simulink model "ADCS_GNC_Real_Simulation"  (R2025a)
settings: Solver=ode4  StartTime=0.0  StopTime=600  FixedStep=dt_sim  RelTol=1e-3
values from neighbouring files (symbols this model uses):
  Area_drag = 1.5    [ADCS_Real_Baseline.m]    (also in ADCS_Real_Baseline_Aerospace_Toolbox.m)
  Cd = 2.2    [ADCS_Real_Baseline.m]    (also in ADCS_Real_Baseline_Aerospace_Toolbox.m)
  cp_cg_offset_drag = [0.05; 0.02; -0.03]    [ADCS_Real_Baseline.m]    (also in ADCS_Real_Baseline_Aerospace_Toolbox.m)
  g0 = 9.80665    [ADCS_Real_Baseline.m]    (also in ADCS_Real_Baseline_Aerospace_Toolbox.m)
  gyro_bias_true = [1e-4; -2e-4; 1.5e-4]    [ADCS_Real_Baseline.m]    (also in ADCS_Real_Baseline_Aerospace_Toolbox.m)
  gyro_noise_sigma = 1e-5    (= 1e-05)    [ADCS_Real_Baseline.m]    (also in ADCS_Real_Baseline_Aerospace_Toolbox.m)
  I_inv = inv(I_tensor)    [ADCS_Real_Baseline.m]    (also in ADCS_Real_Baseline_Aerospace_Toolbox.m)
  I_tensor = diag([I_xx, I_yy, I_zz])    [ADCS_Real_Baseline.m]    (also in ADCS_Real_Baseline_Aerospace_Toolbox.m)
  Kd = diag(diag(2 * zeta * I_tensor * omega_n))    [ADCS_Real_Baseline.m]    (also in ADCS_Real_Baseline_Aerospace_Toolbox.m)
  Kp = diag(diag(I_tensor * omega_n^2))    [ADCS_Real_Baseline.m]    (also in ADCS_Real_Baseline_Aerospace_Toolbox.m)
  mtq_max_dipole = 15.0    (= 15)    [ADCS_Real_Baseline.m]    (also in ADCS_Real_Baseline_Aerospace_Toolbox.m)
  mtq_power_W_per_Am2 = 0.5    [ADCS_Real_Baseline.m]    (also in ADCS_Real_Baseline_Aerospace_Toolbox.m)
  mu_E = 398600.4418    [ADCS_Real_Baseline.m]    (also in ADCS_Real_Baseline_Aerospace_Toolbox.m)
  omega_init = C_BL_init * omega_orb_LVLH    [ADCS_Real_Baseline.m]    (also in ADCS_Real_Baseline_Aerospace_Toolbox.m)
  omega_orb_mag = sqrt(mu_E / r_orbit^3)    [ADCS_Real_Baseline.m]    (also in ADCS_Real_Baseline_Aerospace_Toolbox.m)
  q_init = q_init / norm(q_init)    [ADCS_Real_Baseline.m]    (also in ADCS_Real_Baseline_Aerospace_Toolbox.m)
  q_LVLH_ECI_init = q_LVLH_ECI_init / norm(q_LVLH_ECI_init)    [ADCS_Real_Baseline.m]    (also in ADCS_Real_Baseline_Aerospace_Toolbox.m)
  r_orbit = R_E + h_orbit    (= 7171)    [ADCS_Real_Baseline.m]    (also in ADCS_Real_Baseline_Aerospace_Toolbox.m)
  rho_atm = 1e-13    [ADCS_Real_Baseline.m]    (also in ADCS_Real_Baseline_Aerospace_Toolbox.m)
  rw_max_torque = 0.05    [ADCS_Real_Baseline.m]    (also in ADCS_Real_Baseline_Aerospace_Toolbox.m)
  rw_power_W_per_Nm = 50.0    (= 50)    [ADCS_Real_Baseline.m]    (also in ADCS_Real_Baseline_Aerospace_Toolbox.m)
  st_noise_sigma = 5e-4    (= 0.0005)    [ADCS_Real_Baseline.m]    (also in ADCS_Real_Baseline_Aerospace_Toolbox.m)
  thruster_arm = 0.5    [ADCS_Real_Baseline.m]    (also in ADCS_Real_Baseline_Aerospace_Toolbox.m)
  thruster_Isp = 65.0    (= 65)    [ADCS_Real_Baseline.m]    (also in ADCS_Real_Baseline_Aerospace_Toolbox.m)
  thruster_max_torque = thruster_force * thruster_arm    (= 0.5)    [ADCS_Real_Baseline.m]    (also in ADCS_Real_Baseline_Aerospace_Toolbox.m)
  V_orb = sqrt(mu_E*1e9 / (r_orbit*1e3))    [ADCS_Real_Baseline.m]    (also in ADCS_Real_Baseline_Aerospace_Toolbox.m)
(part 2 of 2)

== matlab function ADCS_GNC_Real_Simulation/Guidance Block ==
  data: t input; q_ref output; omega_orb_mag input; omega_ref output
function [q_ref, omega_ref] = guidance_generator(t, omega_orb_mag)
% =========================================================================
% GUIDANCE & REFERENCE GENERATOR
% =========================================================================
% Purpose:
%   Generate the desired spacecraft attitude and angular velocity.
%
% Mission:
%   Smooth slew from nadir-pointing attitude to an off-nadir attitude.
%
% Reference frames:
%   ECI  = Earth-Centered Inertial frame
%   LVLH = Local Vertical Local Horizontal frame
%   BODY = Spacecraft body frame
%
% Quaternion convention:
%   q = [qw; qx; qy; qz]  (scalar first)
%
% Important convention:
%   q_ref represents the desired BODY orientation with respect to ECI.
%
%   omega_ref is the desired angular velocity of BODY with respect
%   to ECI, but EXPRESSED IN BODY COORDINATES.
%
% =========================================================================
% -------------------------------------------------------------------------
% 1. MANEUVER PARAMETERS
% -------------------------------------------------------------------------
% Time at which the maneuver starts
t_start = 10.0;                         % [s]
% Duration of the maneuver
t_duration = 120.0;                     % [s]
% Final desired attitude with respect to LVLH
roll_target  = deg2rad(30.0);            % [rad]
pitch_target = deg2rad(45.0);            % [rad]
yaw_target   = deg2rad(20.0);            % [rad]
% -------------------------------------------------------------------------
% 2. QUINTIC S-CURVE MANEUVER PROFILE
% -------------------------------------------------------------------------
% alpha goes from 0 to 1.
%
% The quintic polynomial:
%
%   alpha = 10*tau^3 - 15*tau^4 + 6*tau^5
%
% provides:
%   alpha(0) = 0
%   alpha(1) = 1
%   d_alpha(0) = 0
%   d_alpha(1) = 0
%
% Therefore the maneuver starts and ends smoothly.
if t < t_start
    % -------------------------------------------------------------
    % Phase 1: Initial attitude
    % -------------------------------------------------------------
    alpha   = 0.0;
    d_alpha = 0.0;
elseif t <= (t_start + t_duration)
    % -------------------------------------------------------------
    % Phase 2: Slew maneuver
    % -------------------------------------------------------------
    
    % Normalized maneuver time
    tau = (t - t_start) / t_duration;
    % Quintic S-curve
    alpha = 10*tau^3 - 15*tau^4 + 6*tau^5;
    % Derivative of quintic profile
    d_alpha = ...
        (30*tau^2 - 60*tau^3 + 30*tau^4) / t_duration;
else
    % -------------------------------------------------------------
    % Phase 3: Final attitude
    % -------------------------------------------------------------
    alpha   = 1.0;
    d_alpha = 0.0;
end
% -------------------------------------------------------------------------
% 3. CURRENT DESIRED EULER ANGLES
% -------------------------------------------------------------------------
% 3-2-1 / ZYX Euler sequence:
%
%   Roll  = phi
%   Pitch = theta
%   Yaw   = psi
phi   = alpha * roll_target;
theta = alpha * pitch_target;
psi   = alpha * yaw_target;
% -------------------------------------------------------------------------
% 4. EULER ANGLE RATES
% -------------------------------------------------------------------------
% Derivatives of the commanded Euler angles.
d_phi   = d_alpha * roll_target;
d_theta = d_alpha * pitch_target;
d_psi   = d_alpha * yaw_target;
% -------------------------------------------------------------------------
% 5. EULER RATES -> BODY ANGULAR VELOCITY (RIGOROUS 3-2-1 TRANSFORMATION)
% -------------------------------------------------------------------------
% IMPORTANT:
% Euler angle time derivatives (d_phi, d_theta, d_psi) are NOT body rates.
% They must be mapped into the spacecraft Body frame using the 3-2-1 kinematic matrix.
%
% omega_rel is the angular velocity of BODY relative to LVLH,
% expressed in BODY coordinates [rad/s].
omega_rel = [ ...
    d_phi - sin(theta)*d_psi;
    cos(phi)*d_theta + sin(phi)*cos(theta)*d_psi;
   -sin(phi)*d_theta + cos(phi)*cos(theta)*d_psi ];
% -------------------------------------------------------------------------
% 6. EULER ANGLES -> RELATIVE QUATERNION
% -------------------------------------------------------------------------
% Quaternion describing BODY orientation relative to LVLH.
%
% Quaternion convention:
%   q_BL = [qw; qx; qy; qz]
%
% Euler sequence:
%   ZYX / 3-2-1
cy = cos(psi * 0.5);
sy = sin(psi * 0.5);
cp = cos(theta * 0.5);
sp = sin(theta * 0.5);
cr = cos(phi * 0.5);
sr = sin(phi * 0.5);
% Quaternion BODY/LVLH
q_BL = [ ...
    cr*cp*cy + sr*sp*sy;
    sr*cp*cy - cr*sp*sy;
    cr*sp*cy + sr*cp*sy;
    cr*cp*sy - sr*sp*cy ];
% -------------------------------------------------------------------------
% 7. INITIAL LVLH ORIENTATION WITH RESPECT TO ECI
% -------------------------------------------------------------------------
% Initial LVLH-to-ECI orientation.
q_LI_init = [sqrt(2)/2;
             0;
             sqrt(2)/2;
             0];
% -------------------------------------------------------------------------
% 8. ORBITAL ROTATION
% -------------------------------------------------------------------------
% LVLH rotates with the orbit around its Y-axis.
theta_orb = -omega_orb_mag * t;
% Quaternion representing the orbital rotation around LVLH Y-axis
q_orb_rot = [ ...
    cos(theta_orb/2);
    0;
    sin(theta_orb/2);
    0 ];
% -------------------------------------------------------------------------
% 9. CURRENT LVLH ORIENTATION WITH RESPECT TO ECI
% -------------------------------------------------------------------------
% Hamilton quaternion product:
%   q_LI_curr = q_orb_rot * q_LI_init
q_LI_curr = [ ...
    q_orb_rot(1)*q_LI_init(1) ...
        - q_orb_rot(2)*q_LI_init(2) ...
        - q_orb_rot(3)*q_LI_init(3) ...
        - q_orb_rot(4)*q_LI_init(4);
    q_orb_rot(1)*q_LI_init(2) ...
        + q_orb_rot(2)*q_LI_init(1) ...
        + q_orb_rot(3)*q_LI_init(4) ...
        - q_orb_rot(4)*q_LI_init(3);
    q_orb_rot(1)*q_LI_init(3) ...
        - q_orb_rot(2)*q_LI_init(4) ...
        + q_orb_rot(3)*q_LI_init(1) ...
        + q_orb_rot(4)*q_LI_init(2);
    q_orb_rot(1)*q_LI_init(4) ...
        + q_orb_rot(2)*q_LI_init(3) ...
        - q_orb_rot(3)*q_LI_init(2) ...
        + q_orb_rot(4)*q_LI_init(1) ];
% -------------------------------------------------------------------------
% 10. DESIRED ABSOLUTE QUATERNION
% -------------------------------------------------------------------------
% Composition:
%   q_ref = q_BL * q_LI_curr
% Gives the desired BODY attitude with respect to ECI.
q_ref = [ ...
    q_BL(1)*q_LI_curr(1) ...
        - q_BL(2)*q_LI_curr(2) ...
        - q_BL(3)*q_LI_curr(3) ...
        - q_BL(4)*q_LI_curr(4);
    q_BL(1)*q_LI_curr(2) ...
        + q_BL(2)*q_LI_curr(1) ...
        + q_BL(3)*q_LI_curr(4) ...
        - q_BL(4)*q_LI_curr(3);
    q_BL(1)*q_LI_curr(3) ...
        - q_BL(2)*q_LI_curr(4) ...
        + q_BL(3)*q_LI_curr(1) ...
        + q_BL(4)*q_LI_curr(2);
    q_BL(1)*q_LI_curr(4) ...
        + q_BL(2)*q_LI_curr(3) ...
        - q_BL(3)*q_LI_curr(2) ...
        + q_BL(4)*q_LI_curr(1) ];
% -------------------------------------------------------------------------
% 11. DCM: LVLH -> BODY
% -------------------------------------------------------------------------
% Direction Cosine Matrix from LVLH coordinates to BODY coordinates.
C_BL = [ ...
    cp*cy, ...
    cp*sy, ...
   -sp;
    sr*sp*cy - cr*sy, ...
    sr*sp*sy + cr*cy, ...
    sr*cp;
    cr*sp*cy + sr*sy, ...
    cr*sp*sy - sr*cy, ...
    cr*cp ];
% -------------------------------------------------------------------------
% 12. ORBITAL ANGULAR VELOCITY
% -------------------------------------------------------------------------
omega_LVLH = [ ...
    0;
   -omega_orb_mag;
    0 ];
% -------------------------------------------------------------------------
% 13. DESIRED BODY ANGULAR VELOCITY
% -------------------------------------------------------------------------
% omega_ref = omega_body/LVLH (in body) + C_BL * omega_LVLH/ECI (in body)
% IMPORTANT: omega_ref is expressed in BODY coordinates.
omega_ref = omega_rel + C_BL * omega_LVLH;
end

== matlab function ADCS_GNC_Real_Simulation/Sensor Model_1 ==
  settings: updateMethod=DISCRETE
  data: q_true input; q_meas output; omega_true input; st_noise_sigma input; gyro_noise_sigma input; gyro_bias input; omega_meas output
function [q_meas, omega_meas] = sensor_model(q_true, omega_true, st_noise_sigma, gyro_noise_sigma, gyro_bias)
    % =====================================================================
    % SENSOR MODEL (STAR TRACKER & GYROSCOPES)
    % Inputs:
    %   q_true           : 4x1 True attitude quaternion from dynamics
    %   omega_true       : 3x1 True angular velocity from dynamics [rad/s]
    %   st_noise_sigma   : Scalar, Star Tracker noise standard deviation [rad]
    %   gyro_noise_sigma : Scalar, Gyroscope noise standard deviation [rad/s]
    %   gyro_bias        : 3x1 Gyroscope constant thermal drift [rad/s]
    %
    % Outputs:
    %   q_meas           : 4x1 Measured (noisy) quaternion
    %   omega_meas       : 3x1 Measured (noisy) angular velocity
    % =====================================================================

    % 1. GYROSCOPE MODEL (Angular Velocity)
    % Equation: w_meas = w_true + bias + noise
    % We use randn(3,1) to generate normally distributed Gaussian white noise.
    gyro_noise = gyro_noise_sigma * randn(3, 1);
    omega_meas = omega_true + gyro_bias + gyro_noise;

    % 2. STAR TRACKER MODEL (Attitude Quaternion)
    % Instead of adding noise directly to quaternion components (which breaks 
    % its properties), we generate a small random error rotation vector.
    
    % Small angle error on 3 axes [rad]
    err_angles = st_noise_sigma * randn(3, 1);
    
    % Convert small angle error to an error quaternion (Small Angle Approximation)
    % q_err = [1; theta_x/2; theta_y/2; theta_z/2]
    q_err = [1; 0.5 * err_angles(1); 0.5 * err_angles(2); 0.5 * err_angles(3)];
    q_err = q_err / norm(q_err); % Normalize just to be safe
    
    % Apply the error rotation to the true quaternion (Hamilton product)
    % q_meas = q_true * q_err
    qw = q_true(1); qx = q_true(2); qy = q_true(3); qz = q_true(4);
    ew = q_err(1);  ex = q_err(2);  ey = q_err(3);  ez = q_err(4);
    
    q_meas = [ ...
        qw*ew - qx*ex - qy*ey - qz*ez;
        qw*ex + qx*ew + qy*ez - qz*ey;
        qw*ey - qx*ez + qy*ew + qz*ex;
        qw*ez + qx*ey - qy*ex + qz*ew ];
        
    % Final normalization to ensure the controller receives a valid unit quaternion
    q_meas = q_meas / norm(q_meas);
end

== matlab function ADCS_GNC_Real_Simulation/Environment_1 ==
  data: q_BI input; torque_dist output; t input; omega_orb_mag input; q_LVLH_ECI_init input; I_tensor input; mu_E input; r_orbit input; rho_atm input; Cd input; Area_drag input; V_orb input; cp_cg_offset_drag input
function torque_dist = environment_model(q_BI, t, omega_orb_mag, q_LVLH_ECI_init, I_tensor, mu_E, r_orbit, rho_atm, Cd, Area_drag, V_orb, cp_cg_offset_drag)
    % =====================================================================
    % ENVIRONMENTAL DISTURBANCES MODEL
    % Calculates Gravity Gradient and Aerodynamic Drag torques in BODY frame.
    % =====================================================================
    
    % 1. Calculate current LVLH to ECI quaternion (Orbit evolution)
    theta_orb = -omega_orb_mag * t;
    q_orb_rot = [cos(theta_orb/2); 0; sin(theta_orb/2); 0];
    
    % Hamilton product: q_LI_curr = q_orb_rot * q_LVLH_ECI_init
    qw1 = q_orb_rot(1); qx1 = q_orb_rot(2); qy1 = q_orb_rot(3); qz1 = q_orb_rot(4);
    qw2 = q_LVLH_ECI_init(1); qx2 = q_LVLH_ECI_init(2); qy2 = q_LVLH_ECI_init(3); qz2 = q_LVLH_ECI_init(4);
    q_LI_curr = [ ...
        qw1*qw2 - qx1*qx2 - qy1*qy2 - qz1*qz2;
        qw1*qx2 + qx1*qw2 + qy1*qz2 - qz1*qy2;
        qw1*qy2 - qx1*qz2 + qy1*qw2 + qz1*qx2;
        qw1*qz2 + qx1*qy2 - qy1*qx2 + qz1*qw2 ];
        
    % 2. Calculate BODY to LVLH quaternion: q_BL = q_BI * q_LI_curr^(-1)
    q_LI_conj = [q_LI_curr(1); -q_LI_curr(2); -q_LI_curr(3); -q_LI_curr(4)];
    
    qw1 = q_BI(1); qx1 = q_BI(2); qy1 = q_BI(3); qz1 = q_BI(4);
    qw2 = q_LI_conj(1); qx2 = q_LI_conj(2); qy2 = q_LI_conj(3); qz2 = q_LI_conj(4);
    q_BL = [ ...
        qw1*qw2 - qx1*qx2 - qy1*qy2 - qz1*qz2;
        qw1*qx2 + qx1*qw2 + qy1*qz2 - qz1*qy2;
        qw1*qy2 - qx1*qz2 + qy1*qw2 + qz1*qx2;
        qw1*qz2 + qx1*qy2 - qy1*qx2 + qz1*qw2 ];
    q_BL = q_BL / norm(q_BL);
    
    % 3. DCM from LVLH to BODY
    qw = q_BL(1); qx = q_BL(2); qy = q_BL(3); qz = q_BL(4);
    C_BL = [ ...
        1 - 2*(qy^2 + qz^2),     2*(qx*qy + qw*qz),       2*(qx*qz - qw*qy);
        2*(qx*qy - qw*qz),       1 - 2*(qx^2 + qz^2),     2*(qy*qz + qw*qx);
        2*(qx*qz + qw*qy),       2*(qy*qz - qw*qx),       1 - 2*(qx^2 + qy^2) ];
        
    % ---------------------------------------------------------------------
    % A) GRAVITY GRADIENT TORQUE
    % Nadir vector in LVLH is X-axis [1; 0; 0]
    % ---------------------------------------------------------------------
    u_nadir_LVLH = [1; 0; 0];
    u_nadir_BODY = C_BL * u_nadir_LVLH;
    
    % tau_gg = 3 * (mu/r^3) * (u_nadir x I * u_nadir)
    mu_m3 = mu_E * 1e9;         % Convert km^3/s^2 to m^3/s^2
    r_m = r_orbit * 1e3;        % Convert km to m
    tau_gg = 3 * (mu_m3) / (r_m^3) * cross(u_nadir_BODY, I_tensor * u_nadir_BODY);
    
    % ---------------------------------------------------------------------
    % B) AERODYNAMIC DRAG TORQUE
    % Satellite moves along LVLH +Y. So the incoming wind is -Y [0; -1; 0]
    % ---------------------------------------------------------------------
    u_wind_LVLH = [0; -1; 0];
    u_wind_BODY = C_BL * u_wind_LVLH;
    
    % F_drag = 0.5 * rho * Cd * A * V^2 * u_wind
    F_drag_mag = 0.5 * rho_atm * Cd * Area_drag * V_orb^2;
    F_drag_BODY = F_drag_mag * u_wind_BODY;
    
    % tau_drag = offset x F_drag
    tau_drag = cross(cp_cg_offset_drag, F_drag_BODY);
    
    % ---------------------------------------------------------------------
    % TOTAL DISTURBANCE TORQUE
    % ---------------------------------------------------------------------
    torque_dist = tau_gg + tau_drag;
end

== matlab function ADCS_GNC_Real_Simulation/Environment_2 ==
  data: q_BI input; torque_dist output; t input; omega_orb_mag input; q_LVLH_ECI_init input; I_tensor input; mu_E input; r_orbit input; rho_atm input; Cd input; Area_drag input; V_orb input; cp_cg_offset_drag input
function torque_dist = environment_model(q_BI, t, omega_orb_mag, q_LVLH_ECI_init, I_tensor, mu_E, r_orbit, rho_atm, Cd, Area_drag, V_orb, cp_cg_offset_drag)
    % =====================================================================
    % ENVIRONMENTAL DISTURBANCES MODEL
    % Calculates Gravity Gradient and Aerodynamic Drag torques in BODY frame.
    % =====================================================================
    
    % 1. Calculate current LVLH to ECI quaternion (Orbit evolution)
    theta_orb = -omega_orb_mag * t;
    q_orb_rot = [cos(theta_orb/2); 0; sin(theta_orb/2); 0];
    
    % Hamilton product: q_LI_curr = q_orb_rot * q_LVLH_ECI_init
    qw1 = q_orb_rot(1); qx1 = q_orb_rot(2); qy1 = q_orb_rot(3); qz1 = q_orb_rot(4);
    qw2 = q_LVLH_ECI_init(1); qx2 = q_LVLH_ECI_init(2); qy2 = q_LVLH_ECI_init(3); qz2 = q_LVLH_ECI_init(4);
    q_LI_curr = [ ...
        qw1*qw2 - qx1*qx2 - qy1*qy2 - qz1*qz2;
        qw1*qx2 + qx1*qw2 + qy1*qz2 - qz1*qy2;
        qw1*qy2 - qx1*qz2 + qy1*qw2 + qz1*qx2;
        qw1*qz2 + qx1*qy2 - qy1*qx2 + qz1*qw2 ];
        
    % 2. Calculate BODY to LVLH quaternion: q_BL = q_BI * q_LI_curr^(-1)
    q_LI_conj = [q_LI_curr(1); -q_LI_curr(2); -q_LI_curr(3); -q_LI_curr(4)];
    
    qw1 = q_BI(1); qx1 = q_BI(2); qy1 = q_BI(3); qz1 = q_BI(4);
    qw2 = q_LI_conj(1); qx2 = q_LI_conj(2); qy2 = q_LI_conj(3); qz2 = q_LI_conj(4);
    q_BL = [ ...
        qw1*qw2 - qx1*qx2 - qy1*qy2 - qz1*qz2;
        qw1*qx2 + qx1*qw2 + qy1*qz2 - qz1*qy2;
        qw1*qy2 - qx1*qz2 + qy1*qw2 + qz1*qx2;
        qw1*qz2 + qx1*qy2 - qy1*qx2 + qz1*qw2 ];
    q_BL = q_BL / norm(q_BL);
    
    % 3. DCM from LVLH to BODY
    qw = q_BL(1); qx = q_BL(2); qy = q_BL(3); qz = q_BL(4);
    C_BL = [ ...
        1 - 2*(qy^2 + qz^2),     2*(qx*qy + qw*qz),       2*(qx*qz - qw*qy);
        2*(qx*qy - qw*qz),       1 - 2*(qx^2 + qz^2),     2*(qy*qz + qw*qx);
        2*(qx*qz + qw*qy),       2*(qy*qz - qw*qx),       1 - 2*(qx^2 + qy^2) ];
        
    % ---------------------------------------------------------------------
    % A) GRAVITY GRADIENT TORQUE
    % Nadir vector in LVLH is X-axis [1; 0; 0]
    % ---------------------------------------------------------------------
    u_nadir_LVLH = [1; 0; 0];
    u_nadir_BODY = C_BL * u_nadir_LVLH;
    
    % tau_gg = 3 * (mu/r^3) * (u_nadir x I * u_nadir)
    mu_m3 = mu_E * 1e9;         % Convert km^3/s^2 to m^3/s^2
    r_m = r_orbit * 1e3;        % Convert km to m
    tau_gg = 3 * (mu_m3) / (r_m^3) * cross(u_nadir_BODY, I_tensor * u_nadir_BODY);
    
    % ---------------------------------------------------------------------
    % B) AERODYNAMIC DRAG TORQUE
    % Satellite moves along LVLH +Y. So the incoming wind is -Y [0; -1; 0]
    % ---------------------------------------------------------------------
    u_wind_LVLH = [0; -1; 0];
    u_wind_BODY = C_BL * u_wind_LVLH;
    
    % F_drag = 0.5 * rho * Cd * A * V^2 * u_wind
    F_drag_mag = 0.5 * rho_atm * Cd * Area_drag * V_orb^2;
    F_drag_BODY = F_drag_mag * u_wind_BODY;
    
    % tau_drag = offset x F_drag
    tau_drag = cross(cp_cg_offset_drag, F_drag_BODY);
    
    % ---------------------------------------------------------------------
    % TOTAL DISTURBANCE TORQUE
    % ---------------------------------------------------------------------
    torque_dist = tau_gg + tau_drag;
end

== matlab function ADCS_GNC_Real_Simulation/PD Controller_2 ==
  data: q_ref input; torque_cmd output; omega_ref input; q_curr input; omega_curr input; Kp input; Kd input
function torque_cmd = pd_controller(q_ref, omega_ref, q_curr, omega_curr, Kp, Kd)
% =========================================================================
% QUATERNION PD ATTITUDE CONTROLLER
% =========================================================================
% Purpose:
%   Compute the spacecraft control torque required to track the desired
%   attitude and angular velocity.
%
% Inputs:
%   q_ref      : Desired quaternion [qw; qx; qy; qz]
%                BODY attitude with respect to ECI
%
%   omega_ref  : Desired angular velocity [p; q; r]
%                expressed in BODY coordinates
%
%   q_curr     : Current quaternion [qw; qx; qy; qz]
%                BODY attitude with respect to ECI
%
%   omega_curr : Current body angular velocity [p; q; r]
%                expressed in BODY coordinates
%
%   Kp         : Proportional gain matrix
%   Kd         : Derivative gain matrix
%
% Output:
%   torque_cmd : Control torque [Tx; Ty; Tz] in BODY coordinates [Nm]
%
% Quaternion convention:
%   Scalar first: [qw; qx; qy; qz]
%
% =========================================================================


% -------------------------------------------------------------------------
% 1. INITIALIZE OUTPUT
% -------------------------------------------------------------------------

torque_cmd = zeros(3,1);


% -------------------------------------------------------------------------
% 2. NORMALIZE QUATERNIONS
% -------------------------------------------------------------------------
% A valid attitude quaternion must have unit norm.
%
% Normalization also prevents numerical integration errors from
% affecting the attitude error calculation.

q_curr_norm = norm(q_curr);
q_ref_norm  = norm(q_ref);

if q_curr_norm > 1e-12
    q_curr = q_curr / q_curr_norm;
end

if q_ref_norm > 1e-12
    q_ref = q_ref / q_ref_norm;
end


% -------------------------------------------------------------------------
% 3. CURRENT QUATERNION CONJUGATE
% -------------------------------------------------------------------------
% For a unit quaternion:
%
%   q_inverse = conjugate(q)
%
% Therefore:
%
%   q_curr_conj = [qw; -qx; -qy; -qz]

q_curr_conj = [ ...
     q_curr(1);
    -q_curr(2);
    -q_curr(3);
    -q_curr(4) ];


% -------------------------------------------------------------------------
% 4. ATTITUDE ERROR QUATERNION
% -------------------------------------------------------------------------
% We calculate:
%
%   q_err = conjugate(q_curr) * q_ref
%
% With the present convention, the vector part of q_err represents
% the rotation required to move the CURRENT attitude toward the
% REFERENCE attitude, expressed in the current/body coordinates.
%
% This is convenient because the control torque is also expressed
% in BODY coordinates.

% Current quaternion
qc_w = q_curr_conj(1);
qc_x = q_curr_conj(2);
qc_y = q_curr_conj(3);
qc_z = q_curr_conj(4);

% Reference quaternion
qr_w = q_ref(1);
qr_x = q_ref(2);
qr_y = q_ref(3);
qr_z = q_ref(4);


% Hamilton product:
% q_err = q_curr_conj * q_ref

q_err_w = ...
    qc_w*qr_w ...
    - qc_x*qr_x ...
    - qc_y*qr_y ...
    - qc_z*qr_z;

q_err_x = ...
    qc_w*qr_x ...
    + qc_x*qr_w ...
    + qc_y*qr_z ...
    - qc_z*qr_y;

q_err_y = ...
    qc_w*qr_y ...
    - qc_x*qr_z ...
    + qc_y*qr_w ...
    + qc_z*qr_x;

q_err_z = ...
    qc_w*qr_z ...
    + qc_x*qr_y ...
    - qc_y*qr_x ...
    + qc_z*qr_w;


% Vector part of the attitude error
q_err_vec = [ ...
    q_err_x;
    q_err_y;
    q_err_z ];


% -------------------------------------------------------------------------
% 5. SHORTEST-ROTATION PATH
% -------------------------------------------------------------------------
% q and -q represent the same physical attitude.
%
% If the scalar part of the error quaternion is negative, flip the
% vector part so that the controller follows the shortest rotation.

if q_err_w < 0
    q_err_vec = -q_err_vec;
end


% -------------------------------------------------------------------------
% 6. ANGULAR VELOCITY ERROR
% -------------------------------------------------------------------------
% Both omega_curr and omega_ref are expressed in BODY coordinates.
%
% Therefore they can be directly subtracted.

delta_omega = omega_curr - omega_ref;


% -------------------------------------------------------------------------
% 7. QUATERNION PD CONTROL LAW
% -------------------------------------------------------------------------
% Control law:
%
%   torque = Kp * q_error_vector
%            - Kd * angular_velocity_error
%
% The positive proportional sign is consistent with the definition:
%
%   q_err = conjugate(q_curr) * q_ref
%
% A positive q_err vector indicates the direction toward the target.

torque_cmd = Kp * q_err_vec ...
           - Kd * delta_omega;


% -------------------------------------------------------------------------
% 8. OUTPUT
% -------------------------------------------------------------------------
% torque_cmd is expressed in BODY coordinates:
%
%   [Tx; Ty; Tz] [Nm]

end
